simulink model "model1"  (R2019b)
settings: Solver=ode4  StartTime=0.0  StopTime=10.0  FixedStep=0.01  RelTol=1e-3
settings Model: Creator=julie  LastModifiedBy=julie
settings DebuggingCC: UnconnectedInputMsg=none  UnconnectedOutputMsg=none  UnconnectedLineMsg=none  SFMachineParentedDataDiag=error
settings ModelReferenceCC: EnableRefExpFcnMdlSchedulingChecks=off
settings RTWCC: Description=Generic Real-Time Target

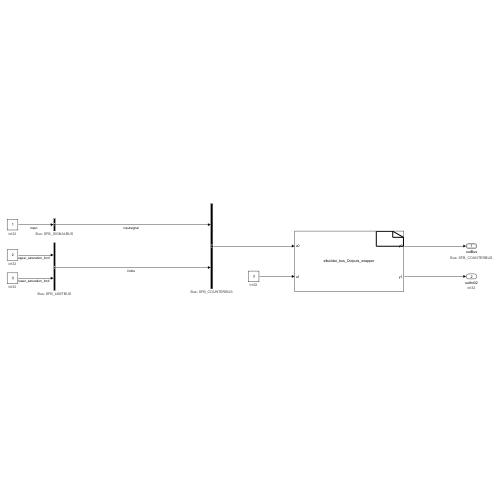
[thumbnail: Simulink's stored preview of the top-level diagram]
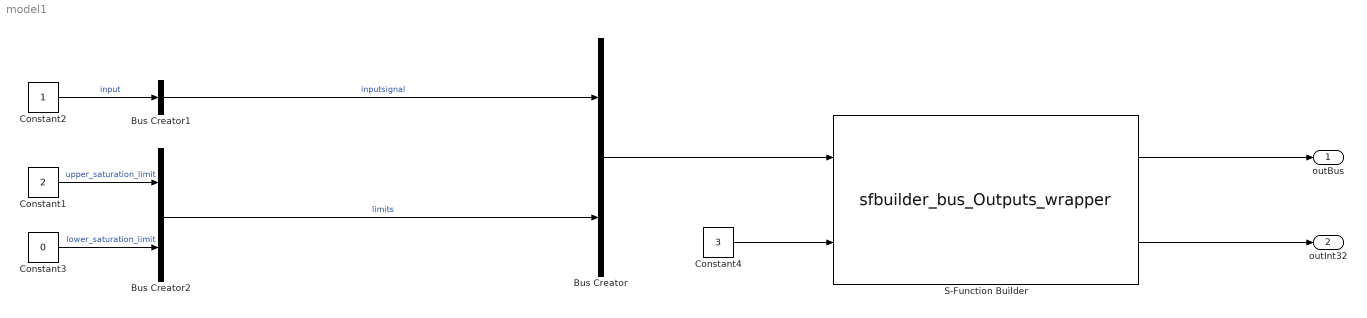
== system model1 ==
  Bus Creator : BusCreator  Inputs=2  OutDataTypeStr=Bus: SFB_COUNTERBUS  NonVirtualBus=on
      settings: AttributesFormatString=%<OutDataTypeStr>
  Bus Creator1 : BusCreator  Inputs=1  OutDataTypeStr=Bus: SFB_SIGNALBUS  NonVirtualBus=on
      settings: AttributesFormatString=%<OutDataTypeStr>
  Bus Creator2 : BusCreator  Inputs=2  OutDataTypeStr=Bus: SFB_LIMITBUS  NonVirtualBus=on
      settings: AttributesFormatString=%<OutDataTypeStr>
  Constant1 : Constant  Value=2  OutDataTypeStr=int32
      settings: AttributesFormatString=%<OutDataTypeStr>
  Constant2 : Constant  OutDataTypeStr=int32
      settings: AttributesFormatString=%<OutDataTypeStr>
  Constant3 : Constant  Value=0  OutDataTypeStr=int32
      settings: AttributesFormatString=%<OutDataTypeStr>
  Constant4 : Constant  Value=3  OutDataTypeStr=int32
      settings: AttributesFormatString=%<OutDataTypeStr>
  S-Function Builder : S-Function  FunctionName=sfbuilder_bus_Outputs_wrapper  SFunctionModules=sfbuilder_bus_Outputs_wrapper_wrapper.c  SFunctionDeploymentMode=off  EnableBusSupport=off  mask(S-Function Builder){}
      mask help: Simulink:masks:SFunctionBuilder_MD
      mask init:
      | val = [[.9  0.75 0.75 1 1 .9 .9 1]',[1 1 0.75 0.75 .9 .9 1 .9]'];try , sys = get_param(gcb,'SfunBuilderFcnName');if isempty(sys), sys = get_param(gcb,'FunctionName'); end,catch, sys = get_param(gcb,'FunctionName'); end
      settings: CopyFcn=set_param(gcbh,'LinkStatus','none')  OpenFcn=sfunctionwizard(gcbh)
      mask Display:
      | plot(val(:,1),val(:,2))
      | disp(sys)
      | port_label('input',1,'u0')
      | port_label('input',2,'u1')
      | port_label('output',1,'y0')
      | port_label('output',2,'y1')
  outBus : Outport  OutDataTypeStr=Bus: SFB_COUNTERBUS  BusOutputAsStruct=on
      settings: AttributesFormatString=%<OutDataTypeStr>
  outInt32 : Outport  Port=2  OutDataTypeStr=int32  PortDimensions=1  BusOutputAsStruct=on
      settings: AttributesFormatString=%<OutDataTypeStr>
  wires:
  Bus Creator/1 -> S-Function Builder/1
  Bus Creator1/1 -> Bus Creator/1  "inputsignal"
  Bus Creator2/1 -> Bus Creator/2  "limits"
  Constant2/1 -> Bus Creator1/1  "input"
  Constant1/1 -> Bus Creator2/1  "upper_saturation_limit"
  Constant3/1 -> Bus Creator2/2  "lower_saturation_limit"
  Constant4/1 -> S-Function Builder/2
  S-Function Builder/1 -> outBus/1
  S-Function Builder/2 -> outInt32/1
